simulink model "conveyer2"  (R2024b)
settings: Solver=VariableStepAuto  StartTime=0.0  StopTime=11  RelTol=1e-3
libraries: fl_lib x27, nesl_utility x15, ee_lib x5, simulink x4

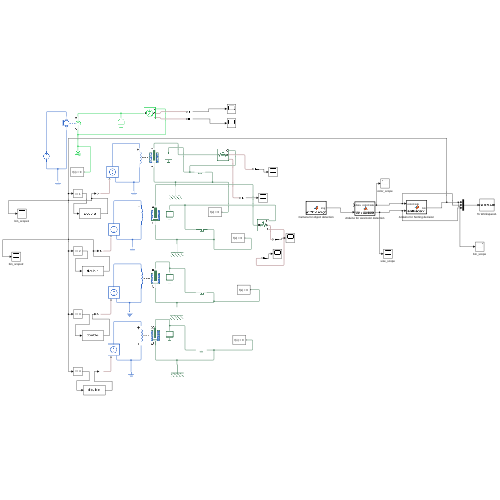
[thumbnail: Simulink's stored preview of the top-level diagram]
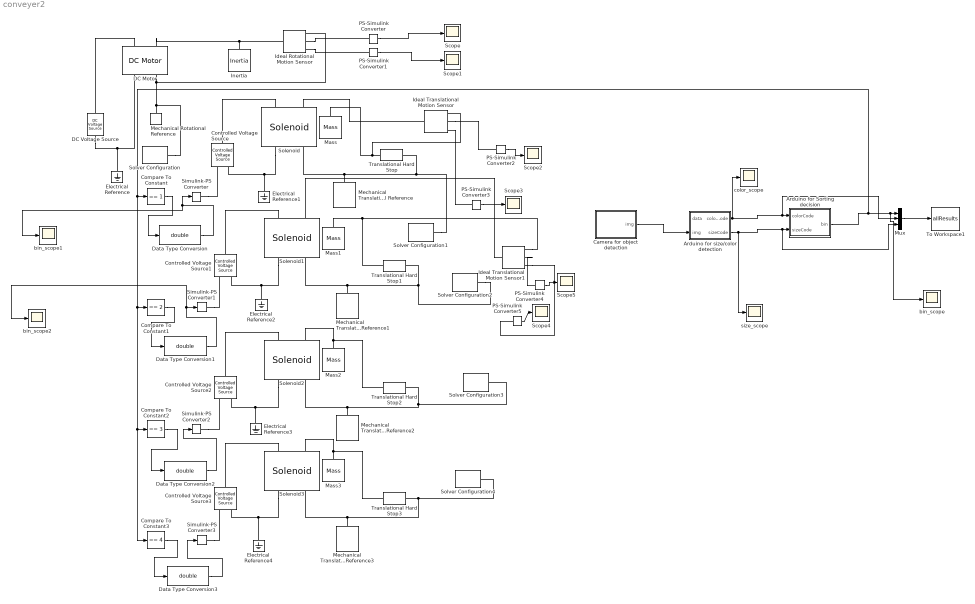
== system conveyer2 ==
  Arduino for Sorting decision : MATLAB Function  TreatAsAtomicUnit=on  SystemSampleTime=1
  Arduino for size/color detection : MATLAB Function  TreatAsAtomicUnit=on  SystemSampleTime=1
  Camera for object detection : MATLAB Function  TreatAsAtomicUnit=on  SystemSampleTime=1
  Compare To Constant : simulink/Logic and Bit Operations/Compare To Constant  relop===  const=1  OutDataTypeStr=uint8  ZeroCross=off
  Compare To Constant1 : simulink/Logic and Bit Operations/Compare To Constant  relop===  const=2  OutDataTypeStr=uint8  ZeroCross=off
  Compare To Constant2 : simulink/Logic and Bit Operations/Compare To Constant  relop===  const=3  OutDataTypeStr=uint8  ZeroCross=off
  Compare To Constant3 : simulink/Logic and Bit Operations/Compare To Constant  relop===  const=4  OutDataTypeStr=uint8  ZeroCross=off
  Controlled Voltage Source{,1..3} (4 alike) : fl_lib/Electrical/Electrical Sources/Controlled Voltage Source
  DC Motor : ee_lib/Electromechanical/Brushed Motors/DC Motor  field_option=ee.enum.field_option.pm  Rf=100 Ohm  Lf=1 H  Laf=0.15 H  If0=0 A  parameterization=ee.enum.dcparam_option.circuit_param  Ra=3.9 Ohm  La=12e-6 H  emf_or_torque=ee.enum.emf_or_torque.kv  Kv=0.072e-3 V/rpm  Ki=6.876e-4 N*m/A  T_stall=0.24e-3 N*m  w_max=19100 rpm  w_rated=15000 rpm  P_rated=0.08 W  V_rated=1.5 V  lam_param=ee.enum.lam_param.damping  i_noload=0 A  V_i_noload=1.5 V  J=0.01 cm^2*g  lam=0 N*m*s/rad  speed0=0 rpm  t_fault_armature=1 s  t_fault_field=1 s  fault_action=simscape.enum.assert.action.none  alpha=3.93e-3 1/K  Tmeas=25 degC  thermal_mass=100 J/K  initial_temperature=25 degC
  DC Voltage Source : fl_lib/Electrical/Electrical Sources/DC Voltage Source  v0=1 V
  Data Type Conversion{,1..3} (4 alike) : DataTypeConversion  OutDataTypeStr=double  SaturateOnIntegerOverflow=off  RndMeth=Floor
  Electrical Reference{,1..4} (5 alike) : fl_lib/Electrical/Electrical Elements/Electrical Reference
  Ideal Rotational Motion Sensor : fl_lib/Mechanical/Mechanical Sensors/Ideal Rotational Motion Sensor  reference=foundation.enum.MeasurementReference.difference  acceleration_port=false  velocity_port=true  position_port=true  wrap_angle=false  offset=0 rad
  Ideal Translational Motion Sensor : fl_lib/Mechanical/Mechanical Sensors/Ideal Translational Motion Sensor  reference=foundation.enum.MeasurementReference.difference  acceleration_port=false  velocity_port=true  position_port=true  offset=0 m
  Ideal Translational Motion Sensor1 : fl_lib/Mechanical/Mechanical Sensors/Ideal Translational Motion Sensor  reference=foundation.enum.MeasurementReference.difference  acceleration_port=false  velocity_port=true  position_port=true  offset=0 m
  Inertia : fl_lib/Mechanical/Rotational Elements/Inertia  inertia=0.01 kg*m^2  num_ports=foundation.enum.numPorts2.one  w_specify=off  w_priority=High  w=0 rad/s  w_nominal_specify=off  w_nominal_value=1  w_nominal_unit=rad/s  t_specify=off  t_priority=None  t=0 N*m  t_nominal_specify=off  t_nominal_value=1  t_nominal_unit=N*m
  Mass{,1..3} (4 alike) : fl_lib/Mechanical/Translational Elements/Mass  mass=1 kg  num_ports=foundation.enum.numPorts2.one  v_specify=off  v_priority=High  v=0 m/s  v_nominal_specify=off  v_nominal_value=1  v_nominal_unit=m/s  f_specify=off  f_priority=None  f=0 N  f_nominal_specify=off  f_nominal_value=1  f_nominal_unit=N
  Mechanical Rotational Reference : fl_lib/Mechanical/Rotational Elements/Mechanical Rotational Reference
  Mechanical Translational Reference{,1..3} (4 alike) : fl_lib/Mechanical/Translational Elements/Mechanical Translational Reference
  Mux : Mux  Inputs=3
  PS-Simulink Converter{,1..5} (6 alike) : nesl_utility/PS-Simulink Converter  PhysicalDomain=network_engine_domain  SubClassName=ps_output  LeftPortType=input  RightPortType=output  PseudoPeriodic=off  Frequencies=[]  VectorFormat=inherit  Unit=inherit  AffineConversion=off
  Scope{,1..5} (6 alike) : Scope
  Simulink-PS Converter{,1..3} (4 alike) : nesl_utility/Simulink-PS Converter  PhysicalDomain=network_engine_domain  SubClassName=ps_input  LeftPortType=input  RightPortType=output  PseudoPeriodic=off  Frequencies=[]  NoiseDistribution=none  NoiseParameters=[]  Unit=1  AffineConversion=off  FilteringAndDerivatives=provide  SimscapeFilterOrder=1  InputFilterTimeConstant=0.001  UdotUserProvided=0
  Solenoid : ee_lib/Electromechanical/Mechatronic Actuators/Solenoid  motionDirection=ee.enum.actuators.solenoidDirection.towards  F12=[7.5, .75] N  X12=[1, 5] mm  Vdc=24 V  Imax=0.05 A  K=200 N/m  Xzero=5 mm  lam=1 N*s/m  Mass=0.05 kg  Xmax=Inf mm  K_endstop=1e6 N/m  D_endstop=500 N*s/m  i_specify=off  i_priority=High  i=0 A  i_nominal_specify=off  i_nominal_value=1  i_nominal_unit=A  x_specify=off  x_priority=High  x=5 mm  x_nominal_specify=off  x_nominal_value=1  x_nominal_unit=mm  vel_specify=off  vel_priority=None  vel=0 mm/s  vel_nominal_specify=off  vel_nominal_value=1  vel_nominal_unit=mm/s  F_specify=off  F_priority=None  F=0 N  F_nominal_specify=off  F_nominal_value=1  F_nominal_unit=N  v_L_specify=off  v_L_priority=None  v_L=0 V  v_L_nominal_specify=off  v_L_nominal_value=1  v_L_nominal_unit=V  magnetic_force_specify=off  magnetic_force_priority=None  magnetic_force=0 N  magnetic_force_nominal_specify=off  magnetic_force_nominal_value=1  magnetic_force_nominal_unit=N  alpha=3.93e-3 1/K  Tmeas=25 degC  thermal_mass=100 J/K  temperature_specify=off  temperature_priority=High  temperature=25 degC  temperature_nominal_specify=off  temperature_nominal_value=1  temperature_nominal_unit=degC  Q_specify=off  Q_priority=None  Q=0 W  Q_nominal_specify=off  Q_nominal_value=1  Q_nominal_unit=W
      settings: InternalSimscapePortConfiguration="{\"Bottom\":[],\"Left\":[{\"id\":\"p\",\"label\":\"+\",\"type\":\"foundation.electrical.electrical\"},{\"id\":\"R\",\"label\":\"R\",\"type\":\"foundation.mechanical.translational.translational\"}],\"Right\":[{\"id\":\"n\",\"label\":\"-\",\"type\":\"foundation.electrical.electrical\"},{\"id\":\"C\",\"label\":\"C\",\"type\":\"foundation.mechanical.translational.translational\"}],\"Top\":[]}"
  Solenoid1 : ee_lib/Electromechanical/Mechatronic Actuators/Solenoid  motionDirection=ee.enum.actuators.solenoidDirection.towards  F12=[7.5, .75] N  X12=[1, 5] mm  Vdc=50 V  Imax=0.05 A  K=200 N/m  Xzero=5 mm  lam=1 N*s/m  Mass=0.05 kg  Xmax=Inf mm  K_endstop=1e6 N/m  D_endstop=500 N*s/m  i_specify=off  i_priority=High  i=0 A  i_nominal_specify=off  i_nominal_value=1  i_nominal_unit=A  x_specify=off  x_priority=High  x=5 mm  x_nominal_specify=off  x_nominal_value=1  x_nominal_unit=mm  vel_specify=off  vel_priority=None  vel=0 mm/s  vel_nominal_specify=off  vel_nominal_value=1  vel_nominal_unit=mm/s  F_specify=off  F_priority=None  F=0 N  F_nominal_specify=off  F_nominal_value=1  F_nominal_unit=N  v_L_specify=off  v_L_priority=None  v_L=0 V  v_L_nominal_specify=off  v_L_nominal_value=1  v_L_nominal_unit=V  magnetic_force_specify=off  magnetic_force_priority=None  magnetic_force=0 N  magnetic_force_nominal_specify=off  magnetic_force_nominal_value=1  magnetic_force_nominal_unit=N  alpha=3.93e-3 1/K  Tmeas=25 degC  thermal_mass=100 J/K  temperature_specify=off  temperature_priority=High  temperature=25 degC  temperature_nominal_specify=off  temperature_nominal_value=1  temperature_nominal_unit=degC  Q_specify=off  Q_priority=None  Q=0 W  Q_nominal_specify=off  Q_nominal_value=1  Q_nominal_unit=W
      settings: InternalSimscapePortConfiguration="{\"Bottom\":[],\"Left\":[{\"id\":\"p\",\"label\":\"+\",\"type\":\"foundation.electrical.electrical\"},{\"id\":\"R\",\"label\":\"R\",\"type\":\"foundation.mechanical.translational.translational\"}],\"Right\":[{\"id\":\"n\",\"label\":\"-\",\"type\":\"foundation.electrical.electrical\"},{\"id\":\"C\",\"label\":\"C\",\"type\":\"foundation.mechanical.translational.translational\"}],\"Top\":[]}"
  Solenoid2 : ee_lib/Electromechanical/Mechatronic Actuators/Solenoid  motionDirection=ee.enum.actuators.solenoidDirection.towards  F12=[7.5, .75] N  X12=[1, 5] mm  Vdc=50 V  Imax=0.05 A  K=200 N/m  Xzero=5 mm  lam=1 N*s/m  Mass=0.05 kg  Xmax=Inf mm  K_endstop=1e6 N/m  D_endstop=500 N*s/m  i_specify=off  i_priority=High  i=0 A  i_nominal_specify=off  i_nominal_value=1  i_nominal_unit=A  x_specify=off  x_priority=High  x=5 mm  x_nominal_specify=off  x_nominal_value=1  x_nominal_unit=mm  vel_specify=off  vel_priority=None  vel=0 mm/s  vel_nominal_specify=off  vel_nominal_value=1  vel_nominal_unit=mm/s  F_specify=off  F_priority=None  F=0 N  F_nominal_specify=off  F_nominal_value=1  F_nominal_unit=N  v_L_specify=off  v_L_priority=None  v_L=0 V  v_L_nominal_specify=off  v_L_nominal_value=1  v_L_nominal_unit=V  magnetic_force_specify=off  magnetic_force_priority=None  magnetic_force=0 N  magnetic_force_nominal_specify=off  magnetic_force_nominal_value=1  magnetic_force_nominal_unit=N  alpha=3.93e-3 1/K  Tmeas=25 degC  thermal_mass=100 J/K  temperature_specify=off  temperature_priority=High  temperature=25 degC  temperature_nominal_specify=off  temperature_nominal_value=1  temperature_nominal_unit=degC  Q_specify=off  Q_priority=None  Q=0 W  Q_nominal_specify=off  Q_nominal_value=1  Q_nominal_unit=W
      settings: InternalSimscapePortConfiguration="{\"Bottom\":[],\"Left\":[{\"id\":\"p\",\"label\":\"+\",\"type\":\"foundation.electrical.electrical\"},{\"id\":\"R\",\"label\":\"R\",\"type\":\"foundation.mechanical.translational.translational\"}],\"Right\":[{\"id\":\"n\",\"label\":\"-\",\"type\":\"foundation.electrical.electrical\"},{\"id\":\"C\",\"label\":\"C\",\"type\":\"foundation.mechanical.translational.translational\"}],\"Top\":[]}"
  Solenoid3 : ee_lib/Electromechanical/Mechatronic Actuators/Solenoid  motionDirection=ee.enum.actuators.solenoidDirection.towards  F12=[7.5, .75] N  X12=[1, 5] mm  Vdc=50 V  Imax=0.05 A  K=200 N/m  Xzero=5 mm  lam=1 N*s/m  Mass=0.05 kg  Xmax=Inf mm  K_endstop=1e6 N/m  D_endstop=500 N*s/m  i_specify=off  i_priority=High  i=0 A  i_nominal_specify=off  i_nominal_value=1  i_nominal_unit=A  x_specify=off  x_priority=High  x=5 mm  x_nominal_specify=off  x_nominal_value=1  x_nominal_unit=mm  vel_specify=off  vel_priority=None  vel=0 mm/s  vel_nominal_specify=off  vel_nominal_value=1  vel_nominal_unit=mm/s  F_specify=off  F_priority=None  F=0 N  F_nominal_specify=off  F_nominal_value=1  F_nominal_unit=N  v_L_specify=off  v_L_priority=None  v_L=0 V  v_L_nominal_specify=off  v_L_nominal_value=1  v_L_nominal_unit=V  magnetic_force_specify=off  magnetic_force_priority=None  magnetic_force=0 N  magnetic_force_nominal_specify=off  magnetic_force_nominal_value=1  magnetic_force_nominal_unit=N  alpha=3.93e-3 1/K  Tmeas=25 degC  thermal_mass=100 J/K  temperature_specify=off  temperature_priority=High  temperature=25 degC  temperature_nominal_specify=off  temperature_nominal_value=1  temperature_nominal_unit=degC  Q_specify=off  Q_priority=None  Q=0 W  Q_nominal_specify=off  Q_nominal_value=1  Q_nominal_unit=W
      settings: InternalSimscapePortConfiguration="{\"Bottom\":[],\"Left\":[{\"id\":\"p\",\"label\":\"+\",\"type\":\"foundation.electrical.electrical\"},{\"id\":\"R\",\"label\":\"R\",\"type\":\"foundation.mechanical.translational.translational\"}],\"Right\":[{\"id\":\"n\",\"label\":\"-\",\"type\":\"foundation.electrical.electrical\"},{\"id\":\"C\",\"label\":\"C\",\"type\":\"foundation.mechanical.translational.translational\"}],\"Top\":[]}"
  Solver Configuration{,1..4} (5 alike) : nesl_utility/Solver Configuration  PhysicalDomain=network_engine_domain  SubClassName=solver  LeftPortType=input  RightPortType=generic  Tones=[]  Harmonics=[]  SimulateNoise=off  Profile=off  UseLocalSampling=off  EnableSwitchedLinearOptims=on  FrequencyDomain=off  UseCCode=off  RelTol=0.001  AbsTol=0.001  MinStep=1e-09  ToWorkspace=off  RevertToSquareIcSolve=off  NumHomotopyIterations=100  PhasorMode=off  PhasorModeNumHarmonics=1  ConsistencySolver=NEWTON_XTOL_AFTER_FTOL  IndexReductionMethod=DerivativeReplacement  DoDC=off  ResidualTolerance=1e-09  ConsistencyTolSource=GLOBAL  ConsistencyAbsTol=0.001  ConsistencyRelTol=0.001  ConsistencyTolFactor=0.001  UseLocalSolver=off  LocalSolverChoice=NE_BACKWARD_EULER_ADVANCER  ResolveIndetEquations=on  FunctionEvalNumThread=1  LocalSolverSampleTime=0.001  DoFixedCost=off  MaxNonlinIter=3  MaxModeIter=2  ComputeImpulses=off  ImpulseIterations=2  LinearAlgebra=auto  LinearAlgebraNumThread=0  EquationFormulation=NE_TIME_EF  DelaysMemoryBudget=1024  AutomaticFiltering=on  FilteringTimeConstant=0.001  PartitionStorageMethod=AS_NEEDED  PartitionMemoryBudget=1024  PartitionMethod=ROBUST  MultibodyUseLocalSolver=off  MultibodyLocalSolverChoice=ODE1  MultibodyLocalSolverSampleTime=0.001
  To Workspace1 : ToWorkspace  VariableName=allResults  SampleTime=-1
  Translational Hard Stop{,1..3} (4 alike) : fl_lib/Mechanical/Translational Elements/Translational Hard Stop  upper_bnd=0.1 m  lower_bnd=-0.1 m  model=simscape.enum.hardstop.smooth  stiff_up=1e6 N/m  stiff_low=1e6 N/m  D_up=150 N*s/m  D_low=150 N*s/m  transition=0.1 mm  coeff_rest=0.7  v_tol=0.001 m/s  f_tol=0.001 N  v_specify=off  v_priority=None  v=0 m/s  v_nominal_specify=off  v_nominal_value=1  v_nominal_unit=m/s  f_specify=off  f_priority=None  f=0 N  f_nominal_specify=off  f_nominal_value=1  f_nominal_unit=N  x_specify=off  x_priority=High  x=0 m  x_nominal_specify=off  x_nominal_value=1  x_nominal_unit=m  M_specify=off  M_priority=None  M=0
  bin_scope : Scope
  bin_scope1 : Scope
  bin_scope2 : Scope
  color_scope : Scope
  size_scope : Scope
  wires:
  PS-Simulink Converter/1 -> Scope/1
  PS-Simulink Converter1/1 -> Scope1/1
  Arduino for size/color detection/2(sizeCode) -> size_scope/1, Mux/3, Arduino for Sorting decision/2(sizeCode)
  Mux/1 -> To Workspace1/1
  Arduino for size/color detection/1(colorCode) -> color_scope/1, Mux/2, Arduino for Sorting decision/1(colorCode)
  Camera for object detection/1(img) -> Arduino for size/color detection/2(img)
  Arduino for Sorting decision/1(bin) -> Compare To Constant3/1, Compare To Constant2/1, Compare To Constant1/1, Compare To Constant/1, bin_scope/1, Mux/1
  Compare To Constant/1 -> Data Type Conversion/1
  Data Type Conversion/1 -> Simulink-PS Converter/1, bin_scope1/1
  Compare To Constant1/1 -> Data Type Conversion1/1
  Data Type Conversion1/1 -> bin_scope2/1, Simulink-PS Converter1/1
  Compare To Constant2/1 -> Data Type Conversion2/1
  Data Type Conversion2/1 -> Simulink-PS Converter2/1
  Compare To Constant3/1 -> Data Type Conversion3/1
  Data Type Conversion3/1 -> Simulink-PS Converter3/1
  PS-Simulink Converter2/1 -> Scope2/1
  PS-Simulink Converter3/1 -> Scope3/1
  PS-Simulink Converter4/1 -> Scope5/1
  PS-Simulink Converter5/1 -> Scope4/1
  connections:
  DC Voltage Source/LConn1 -- DC Motor/LConn1
  DC Voltage Source/RConn1 -- Electrical Reference/LConn1 -- DC Motor/RConn1
  DC Motor/LConn2 -- Ideal Rotational Motion Sensor/LConn1 -- Inertia/LConn1
  DC Motor/RConn2 -- Ideal Rotational Motion Sensor/RConn1 -- Solver Configuration/RConn1 -- Mechanical Rotational Reference/LConn1
  Ideal Rotational Motion Sensor/RConn2 -- PS-Simulink Converter/LConn1
  Ideal Rotational Motion Sensor/RConn3 -- PS-Simulink Converter1/LConn1
  Controlled Voltage Source/LConn1 -- Solenoid/LConn1
  Solenoid/RConn1 -- Controlled Voltage Source/RConn2 -- Electrical Reference1/LConn1
  Mechanical Translational Reference/LConn1 -- Solver Configuration1/RConn1 -- Translational Hard Stop/RConn1 -- Solenoid/RConn2
  Simulink-PS Converter/RConn1 -- Controlled Voltage Source/RConn1
  Translational Hard Stop/LConn1 -- Ideal Translational Motion Sensor/RConn1 -- Mass/LConn1
  Translational Hard Stop1/LConn1 -- Ideal Translational Motion Sensor1/RConn1 -- Mass1/LConn1
  Mechanical Translational Reference1/LConn1 -- Solver Configuration2/RConn1 -- Translational Hard Stop1/RConn1 -- Solenoid1/RConn2
  Controlled Voltage Source1/LConn1 -- Solenoid1/LConn1
  Simulink-PS Converter1/RConn1 -- Controlled Voltage Source1/RConn1
  Solenoid1/RConn1 -- Electrical Reference2/LConn1 -- Controlled Voltage Source1/RConn2
  Solenoid2/LConn2 -- Translational Hard Stop2/LConn1 -- Mass2/LConn1
  Mechanical Translational Reference2/LConn1 -- Translational Hard Stop2/RConn1 -- Solver Configuration3/RConn1 -- Solenoid2/RConn2
  Controlled Voltage Source2/LConn1 -- Solenoid2/LConn1
  Simulink-PS Converter2/RConn1 -- Controlled Voltage Source2/RConn1
  Solenoid2/RConn1 -- Electrical Reference3/LConn1 -- Controlled Voltage Source2/RConn2
  Solenoid3/LConn2 -- Translational Hard Stop3/LConn1 -- Mass3/LConn1
  Mechanical Translational Reference3/LConn1 -- Solver Configuration4/RConn1 -- Translational Hard Stop3/RConn1 -- Solenoid3/RConn2
  Controlled Voltage Source3/LConn1 -- Solenoid3/LConn1
  Simulink-PS Converter3/RConn1 -- Controlled Voltage Source3/RConn1
  Solenoid3/RConn1 -- Controlled Voltage Source3/RConn2 -- Electrical Reference4/LConn1
  Solenoid/LConn2 -- Ideal Translational Motion Sensor/LConn1
  Ideal Translational Motion Sensor/RConn2 -- PS-Simulink Converter2/LConn1
  Ideal Translational Motion Sensor/RConn3 -- PS-Simulink Converter3/LConn1
  Solenoid1/LConn2 -- Ideal Translational Motion Sensor1/LConn1
  Ideal Translational Motion Sensor1/RConn2 -- PS-Simulink Converter4/LConn1
  Ideal Translational Motion Sensor1/RConn3 -- PS-Simulink Converter5/LConn1

== matlab function conveyer2/Camera for object detection ==
  data: img output
function img = getNextImage()
persistent idx imgSet maxIdx
if isempty(idx)
    S = load('imgSet.mat','imgSet'); % Correct way to load
    imgSet = S.imgSet;
    idx = 1;
    maxIdx = numel(imgSet);
end
img = imgSet{idx};
idx = idx + 1;
if idx > maxIdx
    idx = 1;
end

== matlab function conveyer2/Arduino for Sorting decision ==
  data: colorCode input; bin output; sizeCode input
function bin = sortDecision(colorCode, sizeCode)
% Example mapping
% 1=Red, 2=Green, 3=Blue; 1=Small, 2=Large

if colorCode == 1 && sizeCode == 2
    bin = 1;
elseif colorCode == 1 && sizeCode == 1
    bin = 2;
elseif colorCode == 2 && sizeCode == 2
    bin = 3;
elseif colorCode == 2 && sizeCode == 1
    bin = 4;
elseif colorCode == 3 && sizeCode == 2
    bin = 5;
elseif colorCode == 3 && sizeCode == 1
    bin = 6;
else
    bin = 0;
end

== matlab function conveyer2/Arduino for size//color detection ==
  data: data input; img input; colorCode output; sizeCode output
function [colorCode, sizeCode] = detectObject(data, img)
size_thresh = 2000; % Area threshold for small/large

hsv = rgb2hsv(img);

% Color masks
redMask = (hsv(:,:,1)<0.05 | hsv(:,:,1)>0.95) & hsv(:,:,2)>0.5;
greenMask = (hsv(:,:,1)>0.22 & hsv(:,:,1)<0.45) & hsv(:,:,2)>0.5;
blueMask = (hsv(:,:,1)>0.55 & hsv(:,:,1)<0.75) & hsv(:,:,2)>0.5;

masks = {redMask, greenMask, blueMask};
colorCode = 0;
sizeCode = 0;

for c = 1:3
    mask = masks{c};
    mask = bwareaopen(mask, 50);
    props = regionprops(mask, 'Area');
    for k = 1:length(props)
        sz = props(k).Area;
        if sz >= size_thresh
            sizeCode = 2; % 2 = Large
        else
            sizeCode = 1; % 1 = Small
        end
        colorCode = c; % 1=Red, 2=Green, 3=Blue
        return;
    end
end
